simulink model "motor_test"  (R2017a)
settings: Solver=FixedStepDiscrete  StartTime=0.0  StopTime=inf  RelTol=1e-3  EnableMultiTasking=on
PostLoadFcn:
  | PWMFreq = 400;  % 2500ms period
  | Ts = 1/5e3;
libraries: hdlsllib x1
settings Model: DataTypeOverride=Off  ExtModeTrigDuration=100  Creator=skuznick  LastModifiedBy=skuznick
settings SolverCC: PositivePriorityOrder=on
settings DataIOCC: LimitDataPoints=on  SaveFormat=Array  SaveOutput=off  SaveTime=off
settings OptimizationCC: BlockReduction=off  ConditionallyExecuteInputs=off  DefaultParameterBehavior=Inlined  LifeSpan=Inf  MaxStackSize=64
settings DebuggingCC: AlgebraicLoopMsg=error  UnderspecifiedInitializationDetection=Classic  MergeDetectMultiDrivingBlocksExec=none  SingleTaskRateTransMsg=error  StrictBusMsg=ErrorOnBusTreatedAsVector  SFUnexpectedBacktrackingDiag=warning  SFNoUnconditionalDefaultTransitionDiag=warning  SFExecutionAtInitializationDiag=none
settings HardwareCC: ProdBitPerPointer=32  ProdBitPerSizeT=32  ProdBitPerPtrDiffT=32  ProdLargestAtomicFloat=None  ProdIntDivRoundTo=Undefined  ProdEndianess=Unspecified  ProdWordSize=32  ProdHWDeviceType=ASIC/FPGA->ASIC/FPGA  TargetBitPerPointer=64  TargetBitPerSizeT=64  TargetBitPerPtrDiffT=64  TargetLongLongMode=on  TargetIntDivRoundTo=Zero  TargetEndianess=LittleEndian  TargetWordSize=64  TargetHWDeviceType=MATLAB Host  ProdEqTarget=off
settings ModelReferenceCC: PropagateSignalLabelsOutOfModel=off
settings SFSimCC: MATLABDynamicMemAlloc=off
settings RTWCC: SystemTargetFile=ert.tlc  TemplateMakefile=ert_default_tmf  Description=Embedded Coder  GenerateReport=on  RTWVerbose=off  Toolchain=Xilinx Software Development Kit (SDK)  IncludeHyperlinkInReport=on  LaunchReport=on  GenerateTraceInfo=on  GenerateTraceReport=on  GenerateTraceReportSl=on  GenerateTraceReportSf=on  GenerateTraceReportEml=on
settings CodeAppCC: ForceParamTrailComments=on  IgnoreCustomStorageClasses=off  OperatorAnnotations=on  SimulinkDataObjDesc=on  SFDataObjDesc=on  MATLABFcnDesc=on  InsertBlockDesc=on  MATLABSourceComments=on
settings ERTTargetCC: MultiwordLength=2048  SupportVariableSizeSignals=on  ERTCustomFileTemplate=example_file_process.tlc
settings ConfigComp: CovMetricSettings=dw  CovHtmlReporting=on  CovSaveCumulativeToWorkspaceVar=on  CovSaveSingleToWorkspaceVar=on  CovExternalEMLEnable=off

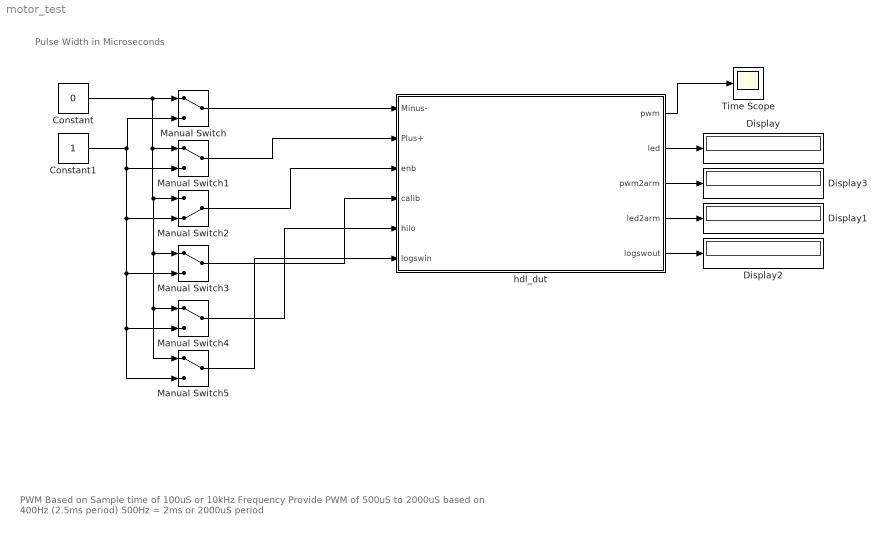
== system motor_test ==
  note: Pulse Width in Microseconds
  note: PWM Based on Sample time of 100uS or 10kHz Frequency
      | Provide PWM of 500uS to 2000uS based on 400Hz (2.5ms period)
      | 500Hz = 2ms or 2000uS period
  Constant : Constant  Value=0  OutDataTypeStr=boolean  SampleTime=-1
  Constant1 : Constant  OutDataTypeStr=boolean  SampleTime=-1
  Display{,1..3} (4 alike) : Display
      Display settings: Format=binary (Stored Integer)
      Display1 settings: Format=binary (Stored Integer)
  Manual Switch{,1,3..5} (5 alike) : ManualSwitch
  Manual Switch2 : ManualSwitch  CurrentSetting=0
  Time Scope : Scope
  hdl_dut : Subsystem  TreatAsAtomicUnit=on  SystemSampleTime=1/fpgaClk  mask{fpgaClk=50e6}
      mask prompts: fpgaClk "FPGA System Clock Freq"
      mask Display:
      | fprintf('FPGA Clock = %d', str2num(get_param(gcb,'fpgaClk')))
      | port_label('input',1,'Minus-')
      | port_label('input',2,'Plus+')
      | port_label('input',3,'Enable')
      | port_label('input',4,'Calib')
      | port_label('input',5,'Lo/Hi')
      | port_label('input',6,'LogSW')
      | port_label('output',1,'PWM')
      | port_label('output',2,'LED')
      | port_label('output',3,'PWM2Arm')
      | port_label('output',4,'LED2Arm')
      | port_label('output',5,'LogSW2Arm')
  wires:
  Constant/1 -> Manual Switch5/1, Manual Switch4/1, Manual Switch3/1, Manual Switch2/1, Manual Switch1/1, Manual Switch/1
  hdl_dut/1(pwm) -> Time Scope/1
  Constant1/1 -> Manual Switch3/2, Manual Switch4/2, Manual Switch5/2, Manual Switch2/2, Manual Switch1/2, Manual Switch/2
  Manual Switch/1 -> hdl_dut/1(Minus-)
  Manual Switch1/1 -> hdl_dut/2(Plus+)
  Manual Switch2/1 -> hdl_dut/3(enb)
  hdl_dut/2(led) -> Display/1
  hdl_dut/5(logswout) -> Display2/1
  hdl_dut/4(led2arm) -> Display1/1
  hdl_dut/3(pwm2arm) -> Display3/1
  Manual Switch3/1 -> hdl_dut/4(calib)
  Manual Switch4/1 -> hdl_dut/5(hilo)
  Manual Switch5/1 -> hdl_dut/6(logswin)

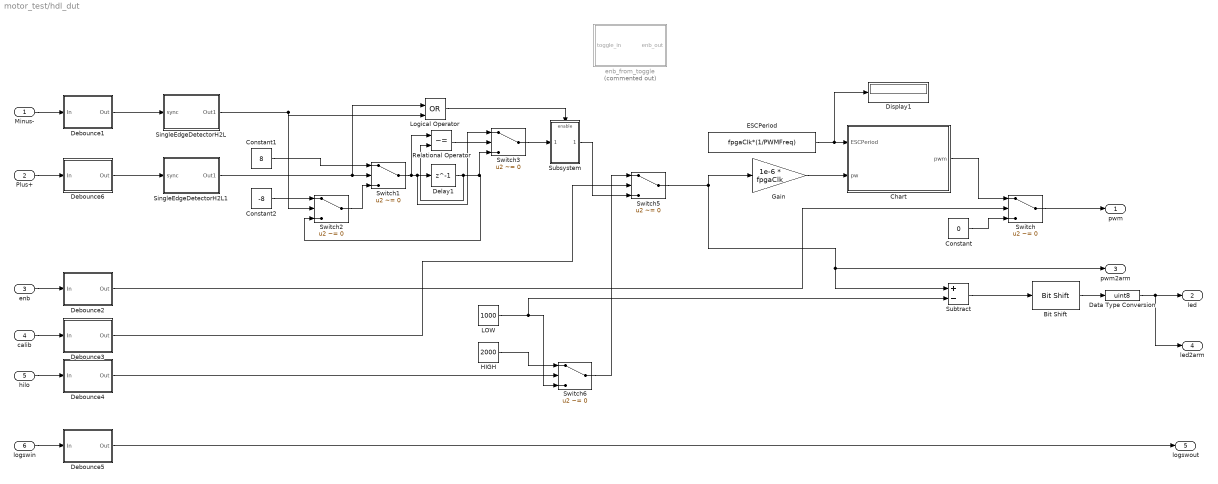
== system motor_test/hdl_dut ==
  Minus- : Inport
  Plus+ : Inport  Port=2
  enb : Inport  Port=3
  calib : Inport  Port=4
  hilo : Inport  Port=5
  logswin : Inport  Port=6
  Bit Shift : hdlsllib/HDL Operations/Bit Shift  mode=Shift Right Arithmetic  N=2
      settings: SourceProductName=HDL Coder  SourceProductBaseCode=HD
  Chart : Stateflow chart  TreatAsAtomicUnit=on
  Constant : Constant  Value=0  OutDataTypeStr=boolean  SampleTime=-1
  Constant1 : Constant  Value=8  OutDataTypeStr=int32  SampleTime=-1
  Constant2 : Constant  Value=-8  OutDataTypeStr=int32  SampleTime=-1
  Data Type Conversion : DataTypeConversion  OutDataTypeStr=uint8
  Debounce1 : Subsystem  TreatAsAtomicUnit=on  mask(Debounce){debounce_count=1}
      mask prompts: debounce_count "Debounce count"
      mask help: Number of consecutive samples before changing states.
  Debounce2 : Subsystem  TreatAsAtomicUnit=on  mask(Debounce){debounce_count=20}
      mask prompts: debounce_count "Debounce count"
      mask help: Number of consecutive samples before changing states.
  Debounce3 : Subsystem  TreatAsAtomicUnit=on  mask(Debounce){debounce_count=20}
      mask prompts: debounce_count "Debounce count"
      mask help: Number of consecutive samples before changing states.
  Debounce4 : Subsystem  TreatAsAtomicUnit=on  mask(Debounce){debounce_count=20}
      mask prompts: debounce_count "Debounce count"
      mask help: Number of consecutive samples before changing states.
  Debounce5 : Subsystem  TreatAsAtomicUnit=on  mask(Debounce){debounce_count=20}
      mask prompts: debounce_count "Debounce count"
      mask help: Number of consecutive samples before changing states.
  Debounce6 : Subsystem  TreatAsAtomicUnit=on  mask(Debounce){debounce_count=1}
      mask prompts: debounce_count "Debounce count"
      mask help: Number of consecutive samples before changing states.
  Delay1 : Delay  DelayLength=1  InitialCondition=0
  Display1 : Display
  ESCPeriod : Constant  Value=fpgaClk*(1/PWMFreq)  OutDataTypeStr=uint32
  Gain : Gain  Gain=1e-6 * fpgaClk  OutDataTypeStr=Inherit: Same as input
  HIGH : Constant  Value=2000  OutDataTypeStr=uint32  SampleTime=-1
  LOW : Constant  Value=1000  OutDataTypeStr=uint32  SampleTime=-1
  Logical Operator : Logic  Operator=OR  IconShape=distinctive  AllPortsSameDT=off  OutDataTypeStr=boolean
  Relational Operator : RelationalOperator  Operator=~=  OutDataTypeStr=boolean  RndMeth=Nearest
  SingleEdgeDetectorH2L : Subsystem  TreatAsAtomicUnit=on
  SingleEdgeDetectorH2L1 : Subsystem  TreatAsAtomicUnit=on
  Subsystem : Subsystem
  Subtract : Sum  Inputs=+-
  Switch{,1..3,5..6} (6 alike) : Switch  Criteria=u2 ~= 0
  enb_from_toggle : Subsystem  Commented=on
  pwm : Outport
  led : Outport  Port=2
  pwm2arm : Outport  Port=3
  led2arm : Outport  Port=4
  logswout : Outport  Port=5
  wires:
  Gain/1 -> Chart/2(pw)
  ESCPeriod/1 -> Display1/1, Chart/1(ESCPeriod)
  enb/1 -> Debounce2/1(In)
  Switch/1 -> pwm/1
  Chart/1(pwm) -> Switch/1
  Constant/1 -> Switch/3
  Minus-/1 -> Debounce1/1(In)
  Plus+/1 -> Debounce6/1(In)
  Constant1/1 -> Switch1/1
  Logical Operator/1 -> Subsystem/Enable
  Switch1/1 -> Relational Operator/1, Switch3/1, Delay1/1
  Switch2/1 -> Switch1/3
  Constant2/1 -> Switch2/1
  SingleEdgeDetectorH2L1/1(Out1) -> Switch1/2, Logical Operator/1
  SingleEdgeDetectorH2L/1(Out1) -> Logical Operator/2, Switch2/2
  Debounce6/1(Out) -> SingleEdgeDetectorH2L1/1(sync)
  Debounce1/1(Out) -> SingleEdgeDetectorH2L/1(sync)
  Debounce2/1(Out) -> Switch/2
  LOW/1 -> Switch6/3, Subtract/2
  Switch6/1 -> Switch5/1
  calib/1 -> Debounce3/1(In)
  Switch5/1 -> pwm2arm/1, Subtract/1, Gain/1
  hilo/1 -> Debounce4/1(In)
  Debounce3/1(Out) -> Switch5/2
  Debounce4/1(Out) -> Switch6/2
  Subtract/1 -> Bit Shift/1
  Bit Shift/1 -> Data Type Conversion/1
  Data Type Conversion/1 -> led2arm/1, led/1
  logswin/1 -> Debounce5/1(In)
  Debounce5/1(Out) -> logswout/1
  HIGH/1 -> Switch6/1
  Subsystem/1(Out1) -> Switch5/3
  Delay1/1 -> Relational Operator/2, Switch3/3, Switch2/3
  Relational Operator/1 -> Switch3/2
  Switch3/1 -> Subsystem/1(In1)

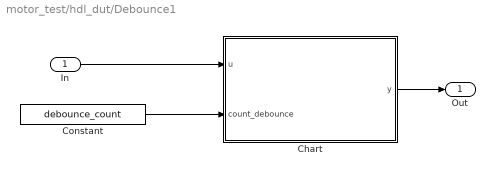
== system motor_test/hdl_dut/Debounce1 ==
  In : Inport
  Chart : Stateflow chart  TreatAsAtomicUnit=on
  Constant : Constant  Value=debounce_count  OutDataTypeStr=uint8  SampleTime=-1
  Out : Outport
  wires:
  In/1 -> Chart/1(u)
  Chart/1(y) -> Out/1
  Constant/1 -> Chart/2(count_debounce)

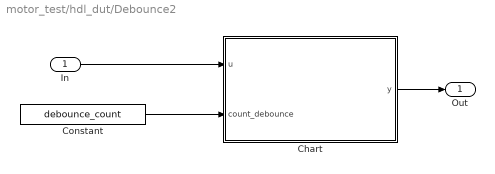
== system motor_test/hdl_dut/Debounce2 ==
  In : Inport
  Chart : Stateflow chart  TreatAsAtomicUnit=on
  Constant : Constant  Value=debounce_count  OutDataTypeStr=uint8  SampleTime=-1
  Out : Outport
  wires:
  In/1 -> Chart/1(u)
  Chart/1(y) -> Out/1
  Constant/1 -> Chart/2(count_debounce)

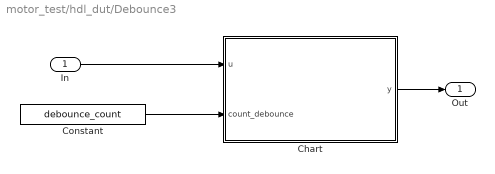
== system motor_test/hdl_dut/Debounce3 ==
  In : Inport
  Chart : Stateflow chart  TreatAsAtomicUnit=on
  Constant : Constant  Value=debounce_count  OutDataTypeStr=uint8  SampleTime=-1
  Out : Outport
  wires:
  Constant/1 -> Chart/2(count_debounce)
  Chart/1(y) -> Out/1
  In/1 -> Chart/1(u)

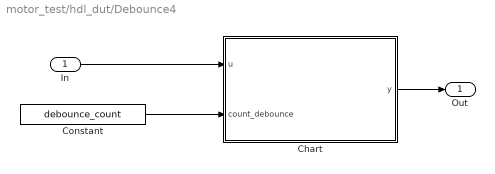
== system motor_test/hdl_dut/Debounce4 ==
  In : Inport
  Chart : Stateflow chart  TreatAsAtomicUnit=on
  Constant : Constant  Value=debounce_count  OutDataTypeStr=uint8  SampleTime=-1
  Out : Outport
  wires:
  In/1 -> Chart/1(u)
  Chart/1(y) -> Out/1
  Constant/1 -> Chart/2(count_debounce)

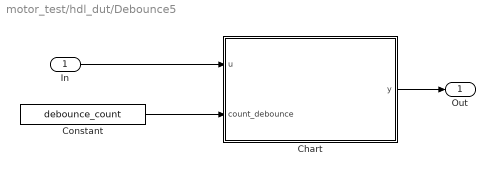
== system motor_test/hdl_dut/Debounce5 ==
  In : Inport
  Chart : Stateflow chart  TreatAsAtomicUnit=on
  Constant : Constant  Value=debounce_count  OutDataTypeStr=uint8  SampleTime=-1
  Out : Outport
  wires:
  Constant/1 -> Chart/2(count_debounce)
  Chart/1(y) -> Out/1
  In/1 -> Chart/1(u)

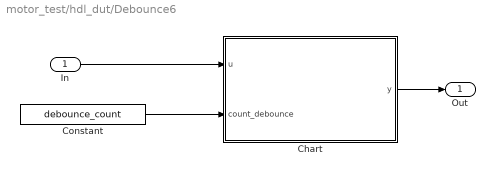
== system motor_test/hdl_dut/Debounce6 ==
  In : Inport
  Chart : Stateflow chart  TreatAsAtomicUnit=on
  Constant : Constant  Value=debounce_count  OutDataTypeStr=uint8  SampleTime=-1
  Out : Outport
  wires:
  Constant/1 -> Chart/2(count_debounce)
  Chart/1(y) -> Out/1
  In/1 -> Chart/1(u)

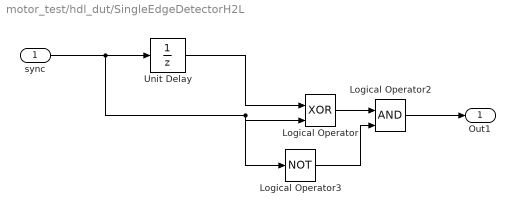
== system motor_test/hdl_dut/SingleEdgeDetectorH2L ==
  sync : Inport  OutDataTypeStr=boolean
  Logical Operator : Logic  Operator=XOR  IconShape=distinctive  AllPortsSameDT=off  OutDataTypeStr=boolean
  Logical Operator2 : Logic  IconShape=distinctive  AllPortsSameDT=off  OutDataTypeStr=boolean
  Logical Operator3 : Logic  Operator=NOT  IconShape=distinctive  AllPortsSameDT=off  OutDataTypeStr=boolean
  Unit Delay : UnitDelay  SampleTime=-1
  Out1 : Outport
  wires:
  Logical Operator3/1 -> Logical Operator2/2
  sync/1 -> Unit Delay/1, Logical Operator3/1, Logical Operator/2
  Logical Operator2/1 -> Out1/1
  Logical Operator/1 -> Logical Operator2/1
  Unit Delay/1 -> Logical Operator/1

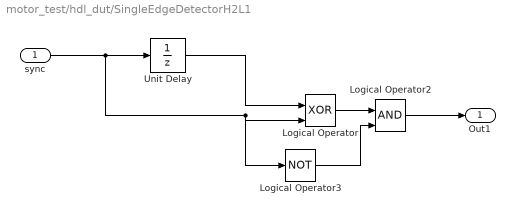
== system motor_test/hdl_dut/SingleEdgeDetectorH2L1 ==
  sync : Inport  OutDataTypeStr=boolean
  Logical Operator : Logic  Operator=XOR  IconShape=distinctive  AllPortsSameDT=off  OutDataTypeStr=boolean
  Logical Operator2 : Logic  IconShape=distinctive  AllPortsSameDT=off  OutDataTypeStr=boolean
  Logical Operator3 : Logic  Operator=NOT  IconShape=distinctive  AllPortsSameDT=off  OutDataTypeStr=boolean
  Unit Delay : UnitDelay  SampleTime=-1
  Out1 : Outport
  wires:
  Unit Delay/1 -> Logical Operator/1
  Logical Operator/1 -> Logical Operator2/1
  Logical Operator2/1 -> Out1/1
  sync/1 -> Logical Operator/2, Logical Operator3/1, Unit Delay/1
  Logical Operator3/1 -> Logical Operator2/2

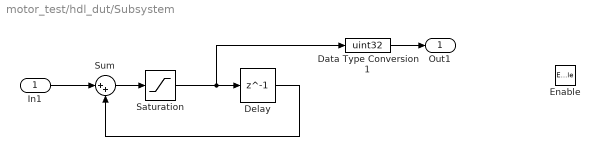
== system motor_test/hdl_dut/Subsystem ==
  In1 : Inport
  Enable : EnablePort
  Data Type Conversion1 : DataTypeConversion  OutDataTypeStr=uint32
  Delay : Delay  DelayLength=1  InitialCondition=1000
  Saturation : Saturate  UpperLimit=2000  LowerLimit=1000
  Sum : Sum  Inputs=|++
  Out1 : Outport  InitialOutput=0
  wires:
  In1/1 -> Sum/1
  Sum/1 -> Saturation/1
  Delay/1 -> Sum/2
  Data Type Conversion1/1 -> Out1/1
  Saturation/1 -> Data Type Conversion1/1, Delay/1

== system motor_test/hdl_dut/enb_from_toggle ==
  toggle_in : Inport
  SingleEdgeDetectorH2L : Subsystem  TreatAsAtomicUnit=on
  toggle : Subsystem
  enb_out : Outport
  wires:
  toggle_in/1 -> SingleEdgeDetectorH2L/1(sync)
  toggle/1(Out1) -> enb_out/1
  SingleEdgeDetectorH2L/1(Out1) -> toggle/Enable

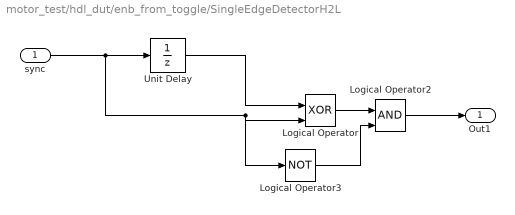
== system motor_test/hdl_dut/enb_from_toggle/SingleEdgeDetectorH2L ==
  sync : Inport  OutDataTypeStr=boolean
  Logical Operator : Logic  Operator=XOR  IconShape=distinctive  AllPortsSameDT=off  OutDataTypeStr=boolean
  Logical Operator2 : Logic  IconShape=distinctive  AllPortsSameDT=off  OutDataTypeStr=boolean
  Logical Operator3 : Logic  Operator=NOT  IconShape=distinctive  AllPortsSameDT=off  OutDataTypeStr=boolean
  Unit Delay : UnitDelay  SampleTime=-1
  Out1 : Outport
  wires:
  Logical Operator3/1 -> Logical Operator2/2
  sync/1 -> Unit Delay/1, Logical Operator3/1, Logical Operator/2
  Logical Operator2/1 -> Out1/1
  Logical Operator/1 -> Logical Operator2/1
  Unit Delay/1 -> Logical Operator/1

== system motor_test/hdl_dut/enb_from_toggle/toggle ==
  Enable : EnablePort
  Delay : Delay  DelayLength=1  InitialCondition=0
  Logical Operator : Logic  Operator=NOT  IconShape=distinctive  AllPortsSameDT=off  OutDataTypeStr=boolean
  Out1 : Outport  InitialOutput=0
  wires:
  Delay/1 -> Out1/1, Logical Operator/1
  Logical Operator/1 -> Delay/1

== stateflow chart motor_test/hdl_dut/Debounce1/Chart ==
  settings: executeAtInitialization=1
  (default) -> (junction 2)
  (junction 2) -> (junction 3) [order 1] : [u == u_n1]
  (junction 2) -> (junction 13) [order 2] : {count = 0;}
  (junction 3) -> (junction 5)
  (junction 5) -> (junction 7) [order 1] : [count >= count_debounce]
  (junction 7) -> (junction 9) : {y = u;}
  (junction 5) -> (junction 11) [order 2] : {count = count + 1;}
  (junction 11) -> (junction 13)
  (junction 9) -> (junction 11)
  (junction 13) -> (junction 17) : {u_n1 = u;}
  data: u input; u_n1 local type(u); y output type(u); count local uint8; count_debounce input

== stateflow chart motor_test/hdl_dut/Debounce6/Chart ==
  settings: executeAtInitialization=1
  (default) -> (junction 2)
  (junction 2) -> (junction 3) [order 1] : [u == u_n1]
  (junction 2) -> (junction 13) [order 2] : {count = 0;}
  (junction 3) -> (junction 5)
  (junction 5) -> (junction 7) [order 1] : [count >= count_debounce]
  (junction 7) -> (junction 9) : {y = u;}
  (junction 5) -> (junction 11) [order 2] : {count = count + 1;}
  (junction 11) -> (junction 13)
  (junction 9) -> (junction 11)
  (junction 13) -> (junction 17) : {u_n1 = u;}
  data: u input; u_n1 local type(u); y output type(u); count local uint8; count_debounce input

== stateflow chart motor_test/hdl_dut/Chart ==
  settings: executeAtInitialization=1
  state on
    entry: cnt = uint32(0);
    pwm = true;
    during: cnt = cnt + 1;
  state off
    entry: pwm = false;
    during: cnt = cnt + 1;
  (default) -> on
  on -> off : [cnt > pw]
  off -> on : [cnt >= ESCPeriod]
  data: ESCPeriod input uint32; pw input uint32; pwm output boolean; cnt local uint32

== stateflow chart motor_test/hdl_dut/Debounce2/Chart ==
  settings: executeAtInitialization=1
  (default) -> (junction 2)
  (junction 2) -> (junction 3) [order 1] : [u == u_n1]
  (junction 2) -> (junction 13) [order 2] : {count = 0;}
  (junction 3) -> (junction 5)
  (junction 5) -> (junction 7) [order 1] : [count >= count_debounce]
  (junction 7) -> (junction 9) : {y = u;}
  (junction 5) -> (junction 11) [order 2] : {count = count + 1;}
  (junction 11) -> (junction 13)
  (junction 9) -> (junction 11)
  (junction 13) -> (junction 17) : {u_n1 = u;}
  data: u input; u_n1 local type(u); y output type(u); count local uint8; count_debounce input

== stateflow chart motor_test/hdl_dut/Debounce3/Chart ==
  settings: executeAtInitialization=1
  (default) -> (junction 2)
  (junction 2) -> (junction 3) [order 1] : [u == u_n1]
  (junction 2) -> (junction 13) [order 2] : {count = 0;}
  (junction 3) -> (junction 5)
  (junction 5) -> (junction 7) [order 1] : [count >= count_debounce]
  (junction 7) -> (junction 9) : {y = u;}
  (junction 5) -> (junction 11) [order 2] : {count = count + 1;}
  (junction 11) -> (junction 13)
  (junction 9) -> (junction 11)
  (junction 13) -> (junction 17) : {u_n1 = u;}
  data: u input; u_n1 local type(u); y output type(u); count local uint8; count_debounce input

== stateflow chart motor_test/hdl_dut/Debounce4/Chart ==
  settings: executeAtInitialization=1
  (default) -> (junction 2)
  (junction 2) -> (junction 3) [order 1] : [u == u_n1]
  (junction 2) -> (junction 13) [order 2] : {count = 0;}
  (junction 3) -> (junction 5)
  (junction 5) -> (junction 7) [order 1] : [count >= count_debounce]
  (junction 7) -> (junction 9) : {y = u;}
  (junction 5) -> (junction 11) [order 2] : {count = count + 1;}
  (junction 11) -> (junction 13)
  (junction 9) -> (junction 11)
  (junction 13) -> (junction 17) : {u_n1 = u;}
  data: u input; u_n1 local type(u); y output type(u); count local uint8; count_debounce input

== stateflow chart motor_test/hdl_dut/Debounce5/Chart ==
  settings: executeAtInitialization=1
  (default) -> (junction 2)
  (junction 2) -> (junction 3) [order 1] : [u == u_n1]
  (junction 2) -> (junction 13) [order 2] : {count = 0;}
  (junction 3) -> (junction 5)
  (junction 5) -> (junction 7) [order 1] : [count >= count_debounce]
  (junction 7) -> (junction 9) : {y = u;}
  (junction 5) -> (junction 11) [order 2] : {count = count + 1;}
  (junction 11) -> (junction 13)
  (junction 9) -> (junction 11)
  (junction 13) -> (junction 17) : {u_n1 = u;}
  data: u input; u_n1 local type(u); y output type(u); count local uint8; count_debounce input
